simulink model "lab1c"  (R2022b)
settings: Solver=FixedStepAuto  StartTime=0.0  StopTime=1.0  FixedStep=1/512  RelTol=1e-3
libraries: dsparch4 x1
settings Model: Creator=simja  LastModifiedBy=simja
settings SolverCC: AutoInsertRateTranBlk=on
settings DataIOCC: ReturnWorkspaceOutputs=off

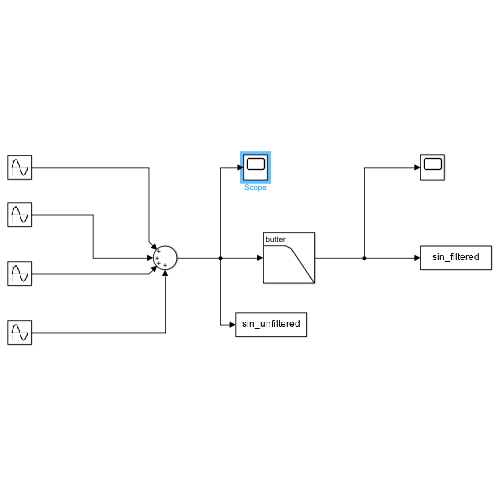
[thumbnail: Simulink's stored preview of the top-level diagram]
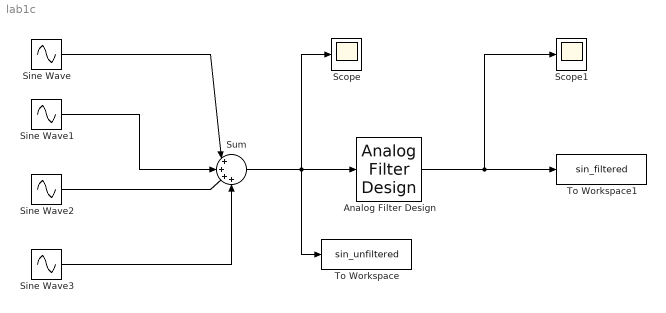
== system lab1c ==
  Analog Filter Design : dsparch4/Analog Filter Design  method=Butterworth  filttype=Lowpass  N=3  Wlo=23*pi*2  Whi=80  Rp=2  Rs=40
  Scope : Scope
  Scope1 : Scope
  Sine Wave : Sin  Amplitude=0.1  Frequency=2*pi*7  SampleTime=0
  Sine Wave1 : Sin  Amplitude=0.1  Frequency=2*pi*18  SampleTime=0
  Sine Wave2 : Sin  Amplitude=0.1  Frequency=2*pi*46  SampleTime=0
  Sine Wave3 : Sin  Amplitude=0.1  Frequency=2*pi*65  SampleTime=0
  Sum : Sum  Inputs=|++++
  To Workspace : ToWorkspace  VariableName=sin_unfiltered  SaveFormat=Structure With Time  SampleTime=-1
  To Workspace1 : ToWorkspace  VariableName=sin_filtered  SaveFormat=Structure With Time  SampleTime=-1
  wires:
  Sine Wave3/1 -> Sum/4
  Sine Wave2/1 -> Sum/3
  Sine Wave1/1 -> Sum/2
  Sine Wave/1 -> Sum/1
  Sum/1 -> Analog Filter Design/1, Scope/1, To Workspace/1
  Analog Filter Design/1 -> Scope1/1, To Workspace1/1
